simulink model "APP_DD1"  (R2018a)
settings: configuration reference "cs_ert" (kept outside this file)
model workspace (MAT data in the model file):
  APP_DD1_DT = 10
values from neighbouring files (symbols this model uses):
  APP_tiSRCHighDefDeb_C = 100.0    [APP_DD1.sldd]
  APP_tiSRCHighOKDeb_C = 100.0    [APP_DD1.sldd]
  APP_tiSRCLowDefDeb_C = 100.0    [APP_DD1.sldd]
  APP_tiSRCLowOKDeb_C = 100.0    [APP_DD1.sldd]
  APP_uRaw1Def_C = 0.0    [APP_DD1.sldd]
  APP_uRaw1SRCHigh_C = 5000.0    [APP_DD1.sldd]
  APP_uRaw1SRCLow_C = 500.0    [APP_DD1.sldd]
libraries: sllib x2
settings Model: DataDictionary=APP_DD1.sldd  Creator=zhoutinglin  LastModifiedBy=zhoutinglin

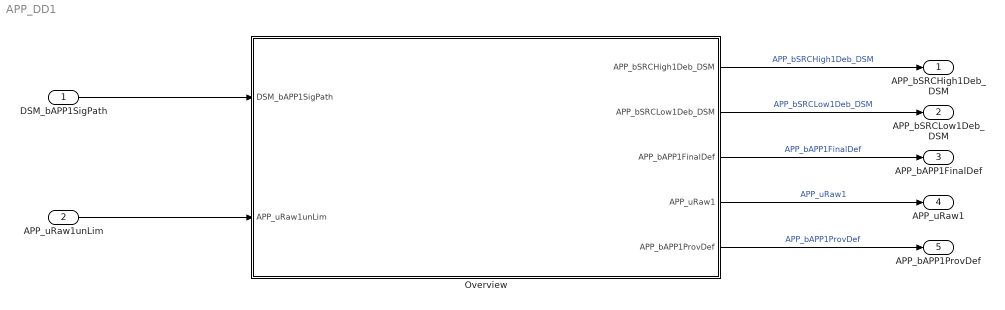
== system APP_DD1 ==
  DSM_bAPP1SigPath : Inport  Description=Acceleration pedal sensor 1 unlimited raw value  OutMin=0  OutMax=1  OutDataTypeStr=boolean  PortDimensions=[1 1]
  APP_uRaw1unLim : Inport  Description=status of FId_APP1SigPath  Port=2  OutMin=0  OutMax=5000  OutDataTypeStr=Volt_mV  PortDimensions=[1 1]
  Overview : Subsystem
  APP_bSRCHigh1Deb_DSM : Outport
  APP_bSRCLow1Deb_DSM : Outport  Port=2
  APP_bAPP1FinalDef : Outport  Port=3
  APP_uRaw1 : Outport  Port=4
  APP_bAPP1ProvDef : Outport  Port=5
  wires:
  DSM_bAPP1SigPath/1 -> Overview/1(DSM_bAPP1SigPath)
  APP_uRaw1unLim/1 -> Overview/2(APP_uRaw1unLim)
  Overview/1(APP_bSRCHigh1Deb_DSM) -> APP_bSRCHigh1Deb_DSM/1  "APP_bSRCHigh1Deb_DSM"
  Overview/2(APP_bSRCLow1Deb_DSM) -> APP_bSRCLow1Deb_DSM/1  "APP_bSRCLow1Deb_DSM"
  Overview/3(APP_bAPP1FinalDef) -> APP_bAPP1FinalDef/1  "APP_bAPP1FinalDef"
  Overview/4(APP_uRaw1) -> APP_uRaw1/1  "APP_uRaw1"
  Overview/5(APP_bAPP1ProvDef) -> APP_bAPP1ProvDef/1  "APP_bAPP1ProvDef"

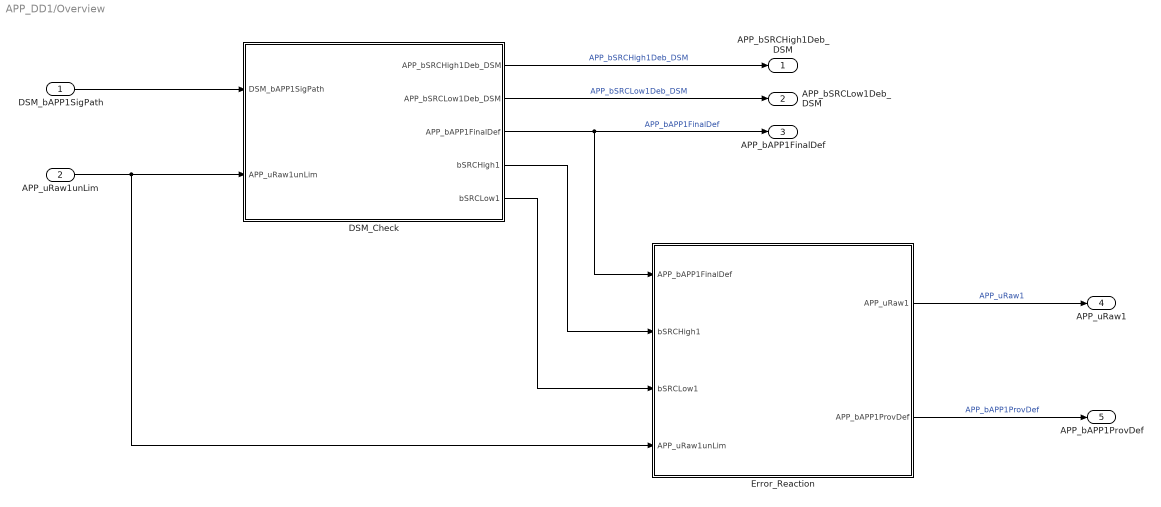
== system APP_DD1/Overview ==
  DSM_bAPP1SigPath : Inport
  APP_uRaw1unLim : Inport  Tag=mv  Port=2
  DSM_Check : Subsystem
  "Error_Reaction " : Subsystem
  APP_bSRCHigh1Deb_DSM : Outport
  APP_bSRCLow1Deb_DSM : Outport  Port=2
  APP_bAPP1FinalDef : Outport  Port=3
  APP_uRaw1 : Outport  Tag=mv  Port=4
  APP_bAPP1ProvDef : Outport  Port=5
  wires:
  "Error_Reaction "/1(APP_uRaw1) -> APP_uRaw1/1  "APP_uRaw1"
  DSM_Check/5(bSRCLow1) -> "Error_Reaction "/3(bSRCLow1)
  DSM_Check/3(APP_bAPP1FinalDef) -> "Error_Reaction "/1(APP_bAPP1FinalDef), APP_bAPP1FinalDef/1  "APP_bAPP1FinalDef"
  DSM_Check/4(bSRCHigh1) -> "Error_Reaction "/2(bSRCHigh1)
  APP_uRaw1unLim/1 -> "Error_Reaction "/4(APP_uRaw1unLim), DSM_Check/2(APP_uRaw1unLim)
  DSM_Check/2(APP_bSRCLow1Deb_DSM) -> APP_bSRCLow1Deb_DSM/1  "APP_bSRCLow1Deb_DSM"
  "Error_Reaction "/2(APP_bAPP1ProvDef) -> APP_bAPP1ProvDef/1  "APP_bAPP1ProvDef"
  DSM_Check/1(APP_bSRCHigh1Deb_DSM) -> APP_bSRCHigh1Deb_DSM/1  "APP_bSRCHigh1Deb_DSM"
  DSM_bAPP1SigPath/1 -> DSM_Check/1(DSM_bAPP1SigPath)

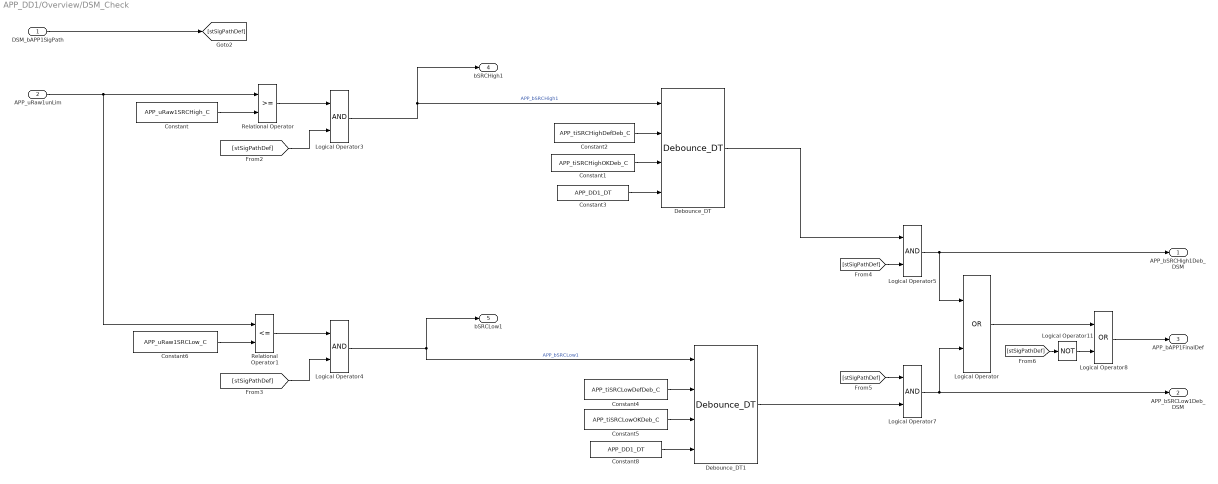
== system APP_DD1/Overview/DSM_Check ==
  DSM_bAPP1SigPath : Inport  Tag=-
  APP_uRaw1unLim : Inport  Tag=mv  Port=2
  Constant : Constant  Value=APP_uRaw1SRCHigh_C
  Constant1 : Constant  Value=APP_tiSRCHighOKDeb_C
  Constant2 : Constant  Value=APP_tiSRCHighDefDeb_C
  Constant3 : Constant  Value=APP_DD1_DT  OutDataTypeStr=Inherit: Inherit via back propagation
  Constant4 : Constant  Value=APP_tiSRCLowDefDeb_C
  Constant5 : Constant  Value=APP_tiSRCLowOKDeb_C
  Constant6 : Constant  Value=APP_uRaw1SRCLow_C
  Constant8 : Constant  Value=APP_DD1_DT  OutDataTypeStr=Inherit: Inherit via back propagation
  Debounce_DT : sllib/Debounce_DT
      settings: SourceProductName=sllib
  Debounce_DT1 : sllib/Debounce_DT
      settings: SourceProductName=sllib
  Logical Operator : Logic  Operator=OR  AllPortsSameDT=off  OutDataTypeStr=boolean
  Logical Operator11 : Logic  Operator=NOT  AllPortsSameDT=off  OutDataTypeStr=boolean
  Logical Operator{3..5,7} (4 alike) : Logic  AllPortsSameDT=off  OutDataTypeStr=boolean
  Logical Operator8 : Logic  Operator=OR  AllPortsSameDT=off  OutDataTypeStr=boolean
  Relational Operator : RelationalOperator  OutDataTypeStr=boolean  RndMeth=Nearest  InputSameDT=on
  Relational Operator1 : RelationalOperator  Operator=<=  OutDataTypeStr=boolean  RndMeth=Nearest  InputSameDT=on
  APP_bSRCHigh1Deb_DSM : Outport  Tag=-
  APP_bSRCLow1Deb_DSM : Outport  Tag=-  Port=2
  APP_bAPP1FinalDef : Outport  Tag=-  Port=3
  bSRCHigh1 : Outport  Port=4
  bSRCLow1 : Outport  Port=5
  wires:
  Debounce_DT/1 -> Logical Operator5/1
  Logical Operator11/1 -> Logical Operator8/2
  Logical Operator8/1 -> APP_bAPP1FinalDef/1
  [stSigPathDef] -> Logical Operator11/1
  Logical Operator/1 -> Logical Operator8/1
  [stSigPathDef] -> Logical Operator7/1
  [stSigPathDef] -> Logical Operator5/2
  [stSigPathDef] -> Logical Operator4/2
  Relational Operator1/1 -> Logical Operator4/1
  [stSigPathDef] -> Logical Operator3/2
  Relational Operator/1 -> Logical Operator3/1
  DSM_bAPP1SigPath/1 -> [stSigPathDef]
  Logical Operator7/1 -> APP_bSRCLow1Deb_DSM/1, Logical Operator/2
  Logical Operator5/1 -> APP_bSRCHigh1Deb_DSM/1, Logical Operator/1
  Logical Operator4/1 -> Debounce_DT1/1, bSRCLow1/1  "APP_bSRCLow1"
  Constant6/1 -> Relational Operator1/2
  Logical Operator3/1 -> Debounce_DT/1, bSRCHigh1/1  "APP_bSRCHigh1"
  Constant/1 -> Relational Operator/2
  APP_uRaw1unLim/1 -> Relational Operator/1, Relational Operator1/1
  Constant8/1 -> Debounce_DT1/4
  Constant3/1 -> Debounce_DT/4
  Constant5/1 -> Debounce_DT1/3
  Constant2/1 -> Debounce_DT/2
  Constant1/1 -> Debounce_DT/3
  Constant4/1 -> Debounce_DT1/2
  Debounce_DT1/1 -> Logical Operator7/2

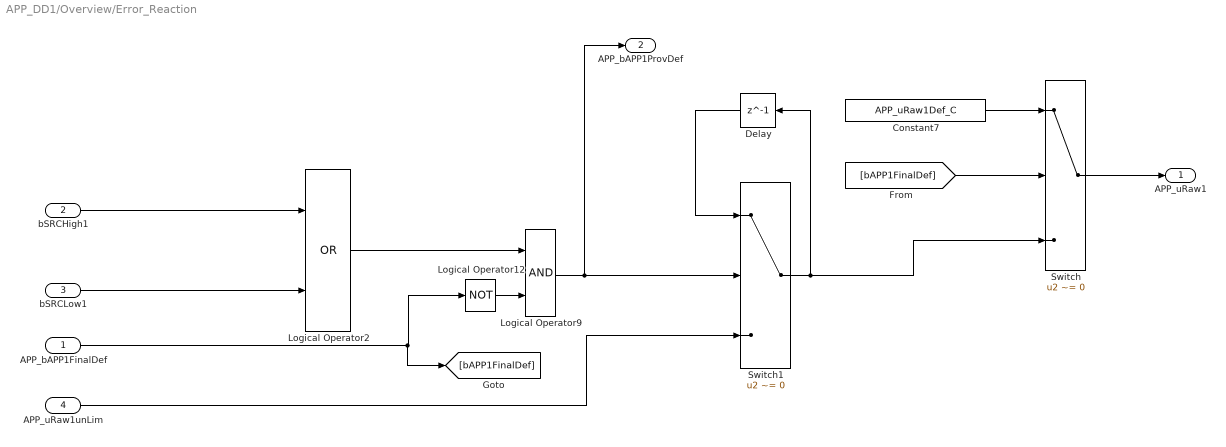
== system APP_DD1/Overview/Error_Reaction  ==
  APP_bAPP1FinalDef : Inport
  bSRCHigh1 : Inport  Port=2
  bSRCLow1 : Inport  Port=3
  APP_uRaw1unLim : Inport  Port=4
  Constant7 : Constant  Value=APP_uRaw1Def_C
  Delay : Delay  DelayLength=1  InitialCondition=0
  Logical Operator12 : Logic  Operator=NOT  AllPortsSameDT=off  OutDataTypeStr=boolean
  Logical Operator2 : Logic  Operator=OR  AllPortsSameDT=off  OutDataTypeStr=boolean
  Logical Operator9 : Logic  AllPortsSameDT=off  OutDataTypeStr=boolean
  Switch : Switch  Criteria=u2 ~= 0
  Switch1 : Switch  Criteria=u2 ~= 0
  APP_uRaw1 : Outport  Tag=mv
  APP_bAPP1ProvDef : Outport  Tag=-  Port=2
  wires:
  Switch/1 -> APP_uRaw1/1
  Delay/1 -> Switch1/1
  Switch1/1 -> Delay/1, Switch/3
  Constant7/1 -> Switch/1
  Logical Operator12/1 -> Logical Operator9/2
  Logical Operator9/1 -> APP_bAPP1ProvDef/1, Switch1/2
  Logical Operator2/1 -> Logical Operator9/1
  bSRCLow1/1 -> Logical Operator2/2
  bSRCHigh1/1 -> Logical Operator2/1
  [bAPP1FinalDef] -> Switch/2
  APP_uRaw1unLim/1 -> Switch1/3
  APP_bAPP1FinalDef/1 -> [bAPP1FinalDef], Logical Operator12/1
